simulink model "LQG_AWBT"  (R2015a)
settings: Solver=ode5  StartTime=0.0  StopTime=14  FixedStep=1e-4  RelTol=1e-3
values from neighbouring files (symbols this model uses):
  Ap = Ap(1:4,1:4)    [main_matlab.m]
  Bp = Bp(1:4,:)    [main_matlab.m]
  Cp = Cp(:,1:4)    [main_matlab.m]
  Hp = Hp(1:4,:)    [main_matlab.m]
  Lambda = X/M    [main_matlab.m]
libraries: cstblocks x2, simulink x1
settings Model: Creator=p4wp4w  LastModifiedBy=p4wp4w

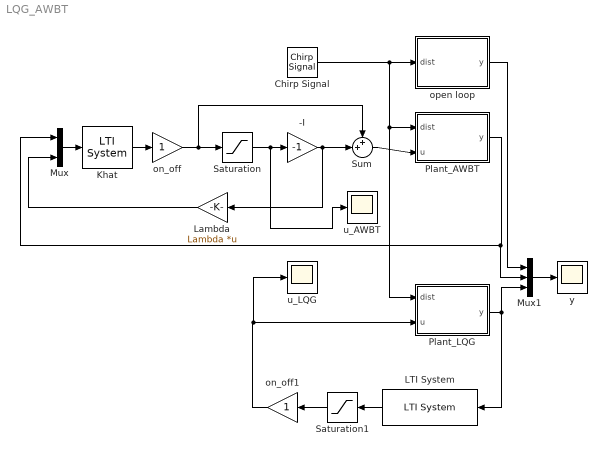
== system LQG_AWBT ==
  -I : Gain  Gain=-1
  Chirp Signal : simulink/Sources/Chirp Signal  f1=0.1  T=14  f2=20
  Khat : cstblocks/LTI System  sys=Khat  IC=[]
  LTI System : cstblocks/LTI System  sys=rlqg  IC=[]
  Lambda : Gain  Gain=Lambda  Multiplication=Matrix(K*u)
  Mux : Mux  Inputs=2
  Mux1 : Mux  Inputs=3
  Plant_AWBT : Subsystem
  Plant_LQG : Subsystem
  Saturation : Saturate  UpperLimit=1.5  LowerLimit=-1.5
  Saturation1 : Saturate  UpperLimit=1.5  LowerLimit=-1.5
  Sum : Sum  Inputs=++|
  on_off : Gain
  on_off1 : Gain
  open loop : Subsystem
  u_AWBT : Scope
      settings: YMin=-0.75  YMax=0.75
  u_LQG : Scope
      settings: SaveName=ScopeData2
  y : Scope
      settings: ShowLegends=on
  wires:
  Mux/1 -> Khat/1
  Plant_AWBT/1(y) -> Mux1/2, Mux/1
  Khat/1 -> on_off/1
  Saturation/1 -> u_AWBT/1, -I/1
  -I/1 -> Sum/2, Lambda/1
  Sum/1 -> Plant_AWBT/2(u)
  on_off/1 -> Sum/1, Saturation/1
  Chirp Signal/1 -> open loop/1(dist), Plant_LQG/1(dist), Plant_AWBT/1(dist)
  Lambda/1 -> Mux/2
  LTI System/1 -> Saturation1/1
  Plant_LQG/1(y) -> Mux1/3, LTI System/1
  Saturation1/1 -> on_off1/1
  Mux1/1 -> y/1
  open loop/1(y) -> Mux1/1
  on_off1/1 -> u_LQG/1, Plant_LQG/2(u)

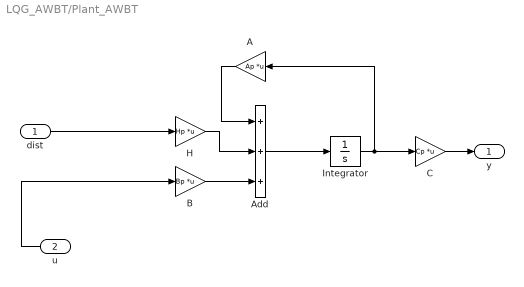
== system LQG_AWBT/Plant_AWBT ==
  dist : Inport
  u : Inport  Port=2
  A : Gain  Gain=Ap  Multiplication=Matrix(K*u)
  Add : Sum  Inputs=+++
  B : Gain  Gain=Bp  Multiplication=Matrix(K*u)
  C : Gain  Gain=Cp  Multiplication=Matrix(K*u)
  H : Gain  Gain=Hp  Multiplication=Matrix(K*u)
  Integrator : Integrator
  y : Outport
  wires:
  Add/1 -> Integrator/1
  H/1 -> Add/2
  A/1 -> Add/1
  dist/1 -> H/1
  C/1 -> y/1
  B/1 -> Add/3
  Integrator/1 -> C/1, A/1
  u/1 -> B/1

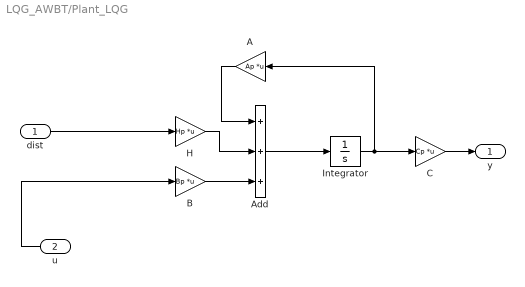
== system LQG_AWBT/Plant_LQG ==
  dist : Inport
  u : Inport  Port=2
  A : Gain  Gain=Ap  Multiplication=Matrix(K*u)
  Add : Sum  Inputs=+++
  B : Gain  Gain=Bp  Multiplication=Matrix(K*u)
  C : Gain  Gain=Cp  Multiplication=Matrix(K*u)
  H : Gain  Gain=Hp  Multiplication=Matrix(K*u)
  Integrator : Integrator
  y : Outport
  wires:
  u/1 -> B/1
  Integrator/1 -> A/1, C/1
  B/1 -> Add/3
  C/1 -> y/1
  dist/1 -> H/1
  A/1 -> Add/1
  H/1 -> Add/2
  Add/1 -> Integrator/1

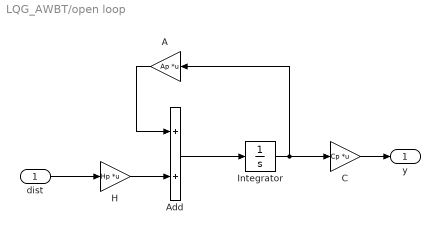
== system LQG_AWBT/open loop ==
  dist : Inport
  A : Gain  Gain=Ap  Multiplication=Matrix(K*u)
  Add : Sum
  C : Gain  Gain=Cp  Multiplication=Matrix(K*u)
  H : Gain  Gain=Hp  Multiplication=Matrix(K*u)
  Integrator : Integrator
  y : Outport
  wires:
  Integrator/1 -> A/1, C/1
  C/1 -> y/1
  dist/1 -> H/1
  A/1 -> Add/1
  H/1 -> Add/2
  Add/1 -> Integrator/1
